simulink model "LAB1_4"  (R2024b)
settings: Solver=FixedStepAuto  StartTime=0.0  StopTime=inf  RelTol=1e-3  EnableMultiTasking=on
libraries: stm32f4xxblockslib x2
settings Model: STM32="{\"AnalogInput\":{\"ID\":\"Test:174\"},\"DigitalPortRead\":{\"ID\":\"Test:183\"}}"  Creator=ASUS  LastModifiedBy=ASUS
settings OptimizationCC: DefaultParameterBehavior=Inlined  EnhancedBackFolding=on  PassReuseOutputArgsAs=Individual arguments  ZeroExternalMemoryAtStartup=off  ZeroInternalMemoryAtStartup=off  MaxStackSize=512  OptimizeBlockOrder=speed  DifferentSizesBufferReuse=on  OptimizationCustomize=off  EfficientTunableParamExpr=on
settings DebuggingCC: ParameterTunabilityLossMsg=error
settings HardwareCC: ProdBitPerPointer=32  ProdBitPerSizeT=32  ProdBitPerPtrDiffT=32  ProdLargestAtomicInteger=Long  ProdLargestAtomicFloat=Double  ProdWordSize=32  ProdLongLongMode=on  ProdHWDeviceType=ARM Compatible->ARM Cortex-M
settings SFSimCC: MATLABDynamicMemAlloc=off
settings RTWCC: Description=Embedded Coder  SystemTargetFile=ert.tlc  HardwareBoard=STM32G4xx Based  TemplateMakefile=ert_default_tmf  Toolchain=GNU Tools for ARM Embedded Processors
settings CodeAppCC: ForceParamTrailComments=on  IgnoreCustomStorageClasses=off  OperatorAnnotations=on  SimulinkDataObjDesc=on  SFDataObjDesc=on  InsertBlockDesc=on
settings ERTTargetCC: TargetLangStandard=C99 (ISO)  CodeReplacementLibrary=ARM Cortex-M  ExtModeTransport=3  ExtModeStaticAlloc=on  ExtModeStaticAllocSize=2048  ExtModeMexFile=ext_xcp  ExtModeIntrfLevel=Level2 - Open

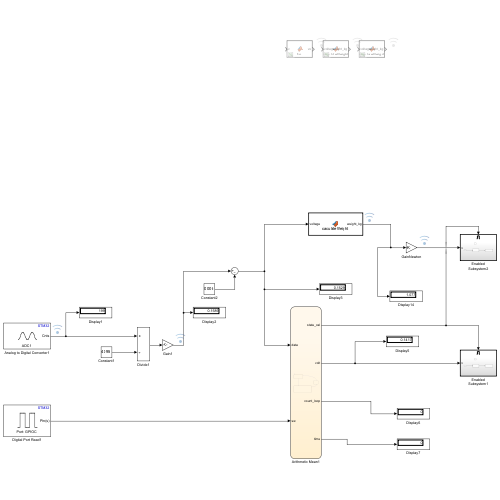
[thumbnail: Simulink's stored preview of the top-level diagram]
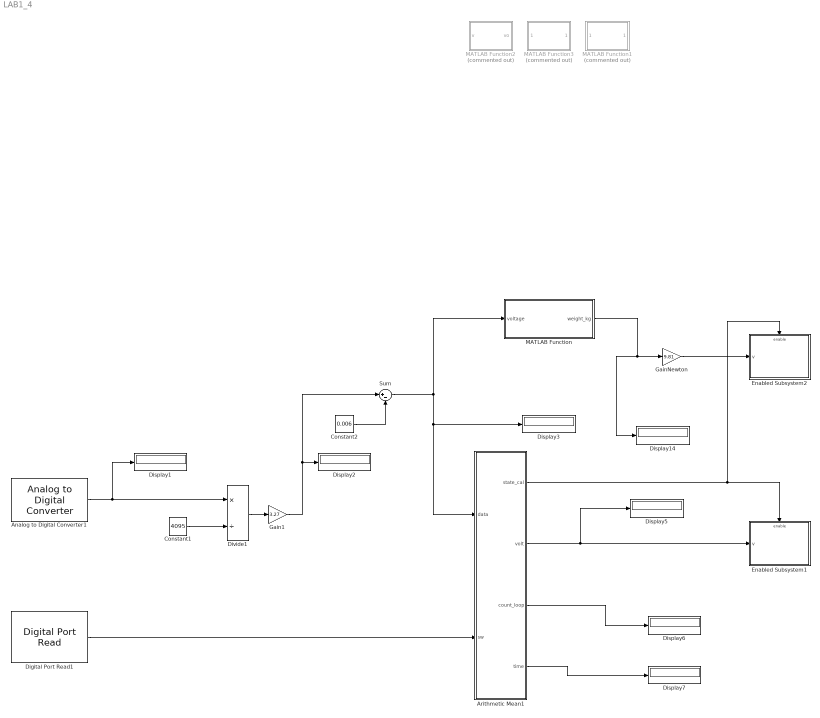
== system LAB1_4 ==
  Analog to Digital Converter1 : stm32f4xxblockslib/Analog to Digital Converter  ADCModule=ADC1  ConversionGroup=Regular  TriggerMode=Trigger and read  NumberOfConversions=1  EnableBufferConv=off  BufferLength=1  OutputStatus=off  SampleTime=-1  EnableSimPort=off  hoistedMaskSrc=ECSoC/ECSimCodegen/Analog to Digital Converter
  Arithmetic Mean1 : Stateflow chart  TreatAsAtomicUnit=on
      settings: PortSchema="{\"entries\":[{\"content\":{\"sides\":[{\"content\":{\"connectorIds\":[\"In2\",\"In1\"]},\"type\":\"ConnectorPlacement.EquallySpacedRectSide\",\"uuid\":\"35d75dd1-7445-4d4a-b8fe-26ed95a9a6b8\"},{\"content\":{\"connectorIds\":[\"Out2\",\"Out4\",\"Out3\",\"Out1\"],\"side\":\"RIGHT\"},\"type\":\"ConnectorPlacement.EquallySpacedRectSide\",\"uuid\":\"b4f8c003-30bf-4716-9840-06738554497d\"},{\"content\":{\"side\":\"TOP\"},\"type\":\"ConnectorPlacement.EquallySpacedRectSide\",\"uuid\":\"cf516399-e2a7-4cee-9ef3-409cd0d6a689\"}]},\"type\":\"ConnectorPlacement.EquallySpacedConnector\",\"uuid\":\"7b96adef-8831-434e-9917-44e023cba094\"}],\"packageUris\":[\"http://schema.mathworks.com/mf0/Connector/R2020b\"],\"version\":\"1.0\"}"
  Constant1 : Constant  Value=4095
  Constant2 : Constant  Value=0.006
  Digital Port Read1 : stm32f4xxblockslib/Digital Port Read  PortName=GPIOC  PinNumber=13  ReadOperation=on  IOAsArray=on  SampleTime=-1  EnableSimPort=off  hoistedMaskSrc=ECSoC/ECSimCodegen/Digital Port Read
      settings: LibrarySourceBlock=stm32g4xxblockslib/Digital Port Read
  Display{1..3,5..7,14} (7 alike) : Display
  Divide1 : Product  Inputs=*/
  Enabled Subsystem1 : Subsystem  TreatAsAtomicUnit=on
  Enabled Subsystem2 : Subsystem  TreatAsAtomicUnit=on
  Gain1 : Gain  Gain=3.27
  GainNewton : Gain  Gain=9.81
  MATLAB Function : MATLAB Function  TreatAsAtomicUnit=on
  MATLAB Function1 : MATLAB Function  Commented=on  TreatAsAtomicUnit=on
  MATLAB Function2 : MATLAB Function  Commented=on  TreatAsAtomicUnit=on
  MATLAB Function3 : MATLAB Function  Commented=on  TreatAsAtomicUnit=on
  Sum : Sum  Inputs=|+-
  wires:
  Divide1/1 -> Gain1/1
  Constant1/1 -> Divide1/2
  Digital Port Read1/1 -> Arithmetic Mean1/1(sw)
  Arithmetic Mean1/1(time) -> Display7/1
  Arithmetic Mean1/2(state_cal) -> Enabled Subsystem2/Enable, Enabled Subsystem1/Enable
  Arithmetic Mean1/3(count_loop) -> Display6/1
  Arithmetic Mean1/4(volt) -> Display5/1, Enabled Subsystem1/1(v)
  Analog to Digital Converter1/1 -> Divide1/1, Display1/1
  MATLAB Function/1(weight_kg) -> GainNewton/1, Display14/1
  Gain1/1 -> Sum/1, Display2/1
  Constant2/1 -> Sum/2
  Sum/1 -> Display3/1, Arithmetic Mean1/2(data), MATLAB Function/1(voltage)
  GainNewton/1 -> Enabled Subsystem2/1(v)

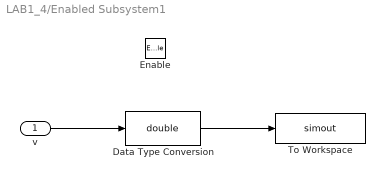
== system LAB1_4/Enabled Subsystem1 ==
  v : Inport
  Enable : EnablePort
  Data Type Conversion : DataTypeConversion  OutDataTypeStr=double  SaturateOnIntegerOverflow=off  RndMeth=Floor
  To Workspace : ToWorkspace  VariableName=simout  SampleTime=-1
      settings: Save2DSignal=2-D array (concatenate along first dimension)
  wires:
  v/1 -> Data Type Conversion/1
  Data Type Conversion/1 -> To Workspace/1

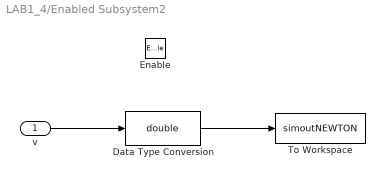
== system LAB1_4/Enabled Subsystem2 ==
  v : Inport
  Enable : EnablePort
  Data Type Conversion : DataTypeConversion  OutDataTypeStr=double  SaturateOnIntegerOverflow=off  RndMeth=Floor
  To Workspace : ToWorkspace  VariableName=simoutNEWTON  SampleTime=-1
      settings: Save2DSignal=2-D array (concatenate along first dimension)
  wires:
  v/1 -> Data Type Conversion/1
  Data Type Conversion/1 -> To Workspace/1

== stateflow chart LAB1_4/Arithmetic Mean1 ==
  state Initial
    volt ;
    time = 0;
    state_cal = 0;
    count_loop=0;
  state StopCount
    entry:
    state_cal = 1
  state CountData
    entry:
    volt = data - data;
    during:
    volt = volt + data
    count_loop=count_loop+1
    time=time+1
    exit:
    volt =volt/1;
  (default) -> Initial
  StopCount -> Initial
  Initial -> CountData : [sw==1]
  CountData -> StopCount : [time>=1]
  data: sw input; data input; time output; state_cal output; count_loop output; volt output

== matlab function LAB1_4/MATLAB Function ==
  data: voltage input; weight_kg output
function weight_kg = calculateWeight(voltage)
    % ตรวจสอบว่า voltage อยู่ในช่วง 0 ถึง 0.142 โวลต์หรือไม่
    if voltage <= 0.142 && voltage >= 0
        % ค่าคงที่จากสมการกำลังสอง
        a = 0.1413;
        b = 0.0027;
        c = - (voltage + 0.0004);  % ปรับค่า c โดยรวมค่า voltage เข้าไป

        % คำนวณค่า discriminant (b^2 - 4ac) เพื่อหาว่ามีรากจริงหรือไม่
        discriminant = b^2 - 4 * a * c;

        % ตรวจสอบว่า discriminant ไม่เป็นค่าลบ (มีรากจริง)
        if discriminant >= 0
            % คำนวณค่ารากทั้งสองจากสมการกำลังสอง
            root1 = (-b + sqrt(discriminant)) / (2 * a);
            root2 = (-b - sqrt(discriminant)) / (2 * a);

            % เลือกใช้รากที่เป็นบวกหรือศูนย์เพื่อให้มีความหมายในเชิงน้ำหนัก
            if root1 >= 0
                weight_kg = root1;
            elseif root2 >= 0
                weight_kg = root2;
            else
                weight_kg = 0;  % หากทั้งสองรากติดลบ กำหนดค่า weight เป็น 0
            end
        else
            % ถ้าไม่มีรากจริง (discriminant < 0) กำหนดค่า weight เป็น 0
            weight_kg = 0;
        end
    elseif voltage <= 0
        weight_kg = 0;
    else
        % หาก voltage อยู่นอกช่วงที่กำหนด ใช้สมการเส้นตรงแทน
        weight_kg = (voltage + 0.1313) / 0.264;
    end
end

== matlab function LAB1_4/MATLAB Function1 ==
  data: voltage input; weight_kg output
function weight_kg = calculateWeight(voltage)
    % ตรวจสอบว่า voltage อยู่ในช่วง 0 ถึง 0.142 โวลต์หรือไม่
    if voltage <= 0.142 && voltage >= 0
        % ค่าคงที่จากสมการกำลังสอง
        a = 0.1413;
        b = 0.0027;
        c = - (voltage + 0.0004);  % ปรับค่า c โดยรวมค่า voltage เข้าไป

        % คำนวณค่า discriminant (b^2 - 4ac) เพื่อหาว่ามีรากจริงหรือไม่
        discriminant = b^2 - 4 * a * c;

        % ตรวจสอบว่า discriminant ไม่เป็นค่าลบ (มีรากจริง)
        if discriminant >= 0
            % คำนวณค่ารากทั้งสองจากสมการกำลังสอง
            root1 = (-b + sqrt(discriminant)) / (2 * a);
            root2 = (-b - sqrt(discriminant)) / (2 * a);

            % เลือกใช้รากที่เป็นบวกหรือศูนย์เพื่อให้มีความหมายในเชิงน้ำหนัก
            if root1 >= 0
                weight_kg = root1;
            elseif root2 >= 0
                weight_kg = root2;
            else
                weight_kg = 0;  % หากทั้งสองรากติดลบ กำหนดค่า weight เป็น 0
            end
        else
            % ถ้าไม่มีรากจริง (discriminant < 0) กำหนดค่า weight เป็น 0
            weight_kg = 0;
        end
    elseif voltage <= 0
        weight_kg = 0;
    else
        % หาก voltage อยู่นอกช่วงที่กำหนด ใช้สมการเส้นตรงแทน
        weight_kg = (voltage + 0.1313) / 0.264;
    end
end

== matlab function LAB1_4/MATLAB Function2 ==
  data: v input; vo output
function vo = fcn(v)
        if v >= 0.006
            vo = v-0.006;  
        else 
            vo = 0 ;
        end

== matlab function LAB1_4/MATLAB Function3 ==
  data: voltage input; weight_kg output
function weight_kg = calculateWeight(voltage)
    % คำนวณน้ำหนักเป็นกิโลกรัม (weight_kg) จากค่าแรงดันไฟฟ้า (voltage)
    
    % กรณีที่ voltage อยู่ในช่วง 0 ถึง 0.142 โวลต์
    if voltage <= 0.142 && voltage >= 0
        % ใช้สมการที่กำหนดสำหรับช่วงแรงดันไฟฟ้านี้
        weight_kg = 2.4949e+03 * (sin(voltage - pi)) - 125.5428 * ((voltage - 10)^2) + 1.2554e+04;
    
    % กรณีที่ voltage น้อยกว่าหรือเท่ากับ 0
    elseif voltage <= 0
        % กำหนด weight_kg เป็น 0
        weight_kg = 0;
    
    % กรณีที่ voltage อยู่นอกช่วงที่กำหนด
    else
        % ใช้สมการเส้นตรงในการประมาณค่า weight_kg
        weight_kg = (voltage + 0.1313) / 0.264;
    end
end
